simulink model "vspu2024_model"  (R2022b)
settings: Solver=ode1  StartTime=0.0  StopTime=25  FixedStep=10^-5  RelTol=1e-3
values from neighbouring files (symbols this model uses):
  a0 = 1    [vspu_params.m]
  a1 = 2    [vspu_params.m]
  a2 = 1    [vspu_params.m]
  a3 = 2    [vspu_params.m]
  a4 = 0.01    [vspu_params.m]
  a5 = 1    [vspu_params.m]
  a6 = 1    [vspu_params.m]
  a7 = 1    [vspu_params.m]
  k = 1    [vspu_params.m]
undefined symbols (not defined in the file or in its folder): adjoint
settings Model: Creator=LastConst  LastModifiedBy=LastConst
settings SolverCC: AlgebraicLoopSolver=TrustRegion
settings DataIOCC: ReturnWorkspaceOutputs=off
settings DebuggingCC: UnconnectedInputMsg=warning  UnconnectedOutputMsg=warning  UnconnectedLineMsg=warning  SFMachineParentedDataDiag=warning  ArithmeticOperatorsInVariantConditions=warning
settings ModelReferenceCC: EnableRefExpFcnMdlSchedulingChecks=on
settings SFSimCC: SimUseLocalCustomCode=off  CustomCodeUndefinedFunction=UseInterfaceOnly
settings RTWCC: RTWUseLocalCustomCode=off
settings CodeAppCC: StateflowObjectComments=on

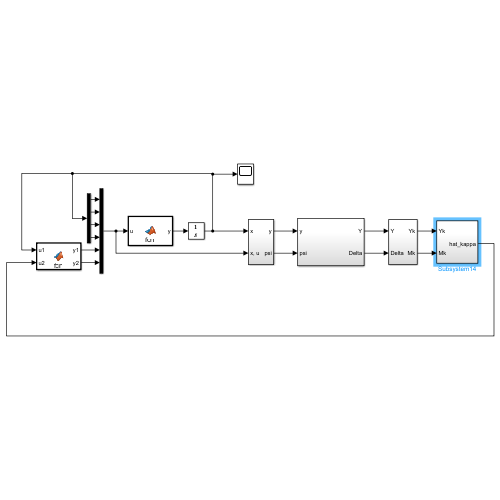
[thumbnail: Simulink's stored preview of the top-level diagram]
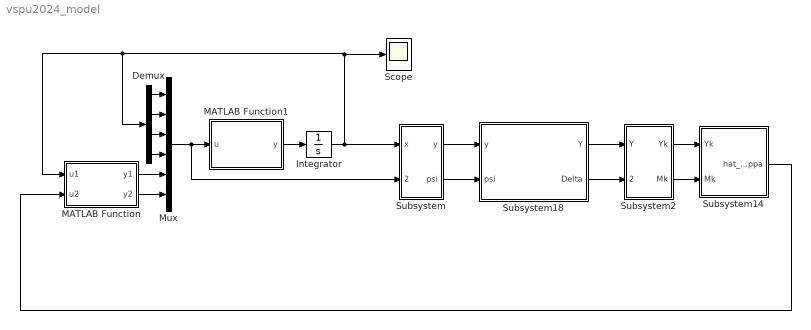
== system vspu2024_model ==
  Demux : Demux
  Integrator : Integrator  InitialCondition=[-1; 1;0.2;-0.2]*100
  MATLAB Function : MATLAB Function  TreatAsAtomicUnit=on
  MATLAB Function1 : MATLAB Function  TreatAsAtomicUnit=on
  Mux : Mux  Inputs=6
  Scope : Scope
  Subsystem : Subsystem
  Subsystem14 : Subsystem
  Subsystem18 : Subsystem
  Subsystem2 : Subsystem
  wires:
  Demux/1 -> Mux/1
  Demux/2 -> Mux/2
  Demux/3 -> Mux/3
  Demux/4 -> Mux/4
  MATLAB Function/2(y2) -> Mux/6
  MATLAB Function/1(y1) -> Mux/5
  Integrator/1 -> Scope/1, MATLAB Function/1(u1), Demux/1, Subsystem/1(x)
  Subsystem14/1(hat_kappa) -> MATLAB Function/2(u2)
  Mux/1 -> MATLAB Function1/1(u), Subsystem/2("x, u")
  MATLAB Function1/1(y) -> Integrator/1
  Subsystem2/1(Yk) -> Subsystem14/1(Yk)
  Subsystem2/2(Mk) -> Subsystem14/2(Mk)
  Subsystem/1(y) -> Subsystem18/1(y)
  Subsystem/2(psi) -> Subsystem18/2(psi)
  Subsystem18/1(Y) -> Subsystem2/1(Y)
  Subsystem18/2(Delta) -> Subsystem2/2(Delta)

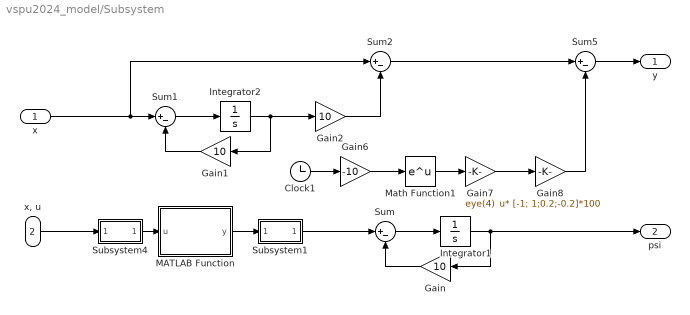
== system vspu2024_model/Subsystem ==
  x : Inport
  "x, u" : Inport  Port=2
  Clock1 : Clock
  Gain : Gain  Gain=10
  Gain1 : Gain  Gain=10
  Gain2 : Gain  Gain=10
  Gain6 : Gain  Gain=-10
  Gain7 : Gain  Gain=eye(4)
  Gain8 : Gain  Gain=[-1; 1;0.2;-0.2]*100  Multiplication=Matrix(u*K)
  Integrator1 : Integrator
  Integrator2 : Integrator
  MATLAB Function : MATLAB Function  TreatAsAtomicUnit=on
  Math Function1 : Math  SignedPower=on
  Subsystem1 : Subsystem
  Subsystem4 : Subsystem
  Sum{,1..2,5} (4 alike) : Sum  Inputs=|+-
  y : Outport
  psi : Outport  Port=2
  wires:
  MATLAB Function/1(y) -> Subsystem1/1(In1)
  Gain2/1 -> Sum2/2
  Sum/1 -> Integrator1/1
  Gain/1 -> Sum/2
  Sum1/1 -> Integrator2/1
  Integrator2/1 -> Gain2/1, Gain1/1
  Gain1/1 -> Sum1/2
  x/1 -> Sum2/1, Sum1/1
  "x, u"/1 -> Subsystem4/1(In1)
  Integrator1/1 -> psi/1, Gain/1
  Subsystem4/1(Out1) -> MATLAB Function/1(u)
  Subsystem1/1(Out1) -> Sum/1
  Gain6/1 -> Math Function1/1
  Clock1/1 -> Gain6/1
  Math Function1/1 -> Gain7/1
  Gain7/1 -> Gain8/1
  Gain8/1 -> Sum5/2
  Sum2/1 -> Sum5/1
  Sum5/1 -> y/1

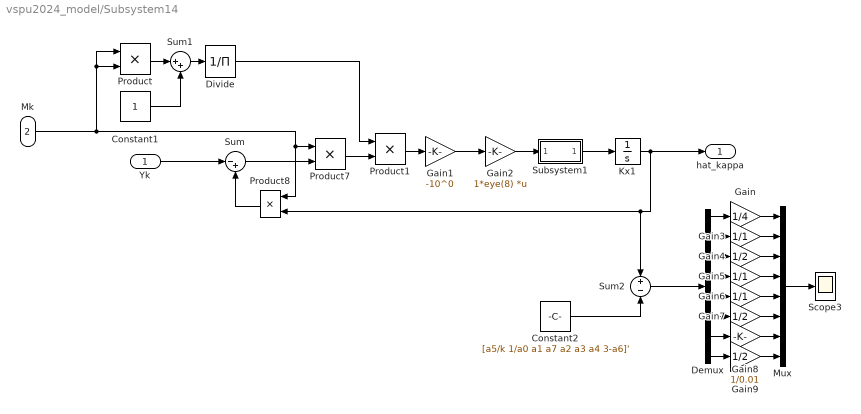
== system vspu2024_model/Subsystem14 ==
  Yk : Inport
  Mk : Inport  Port=2
  Constant1 : Constant
  Constant2 : Constant  Value=[a5/k 1/a0 a1 a7 a2 a3 a4 3-a6]'
  Demux : Demux  Outputs=8
  Divide : Product  Inputs=/
  Gain : Gain  Gain=1/4
  Gain1 : Gain  Gain=-10^0
  Gain2 : Gain  Gain=1*eye(8)  Multiplication=Matrix(K*u)
  Gain3 : Gain  Gain=1/1
  Gain4 : Gain  Gain=1/2
  Gain5 : Gain  Gain=1/1
  Gain6 : Gain  Gain=1/1
  Gain7 : Gain  Gain=1/2
  Gain8 : Gain  Gain=1/0.01
  Gain9 : Gain  Gain=1/2
  Kx1 : Integrator  InitialCondition=[5 0 0 0 0 0 0 0]'
  Mux : Mux  Inputs=8
  Product{,1,7..8} (4 alike) : Product
  Scope3 : Scope
  Subsystem1 : Subsystem
  Sum : Sum  Inputs=|-+
  Sum1 : Sum  Inputs=|++
  Sum2 : Sum  Inputs=+-
  hat_kappa : Outport
  wires:
  Product8/1 -> Sum/2
  Product7/1 -> Product1/2
  Sum/1 -> Product7/2
  Divide/1 -> Product1/1
  Subsystem1/1(Out1) -> Kx1/1
  Product1/1 -> Gain1/1
  Yk/1 -> Sum/1
  Gain2/1 -> Subsystem1/1(In1)
  Mk/1 -> Product/1, Product/2, Product7/1, Product8/1
  Kx1/1 -> hat_kappa/1, Sum2/1, Product8/2
  Constant2/1 -> Sum2/2
  Sum1/1 -> Divide/1
  Product/1 -> Sum1/1
  Constant1/1 -> Sum1/2
  Gain1/1 -> Gain2/1
  Sum2/1 -> Demux/1
  Mux/1 -> Scope3/1
  Demux/3 -> Gain4/1
  Demux/1 -> Gain/1
  Demux/2 -> Gain3/1
  Demux/4 -> Gain5/1
  Demux/5 -> Gain6/1
  Demux/6 -> Gain7/1
  Demux/7 -> Gain8/1
  Demux/8 -> Gain9/1
  Gain/1 -> Mux/1
  Gain3/1 -> Mux/2
  Gain4/1 -> Mux/3
  Gain5/1 -> Mux/4
  Gain6/1 -> Mux/5
  Gain7/1 -> Mux/6
  Gain8/1 -> Mux/7
  Gain9/1 -> Mux/8

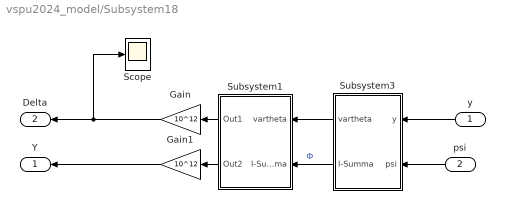
== system vspu2024_model/Subsystem18 ==
  y : Inport
  psi : Inport  Port=2
  Gain : Gain  Gain=10^12
  Gain1 : Gain  Gain=10^12
  Scope : Scope
  Subsystem1 : Subsystem
  Subsystem3 : Subsystem
  Y : Outport
  Delta : Outport  Port=2
  wires:
  Subsystem1/2(Out2) -> Gain1/1
  y/1 -> Subsystem3/1(y)
  Subsystem3/2(I-Summa) -> Subsystem1/2(I-Summa)  "Ф"
  Gain/1 -> Scope/1, Delta/1
  Subsystem3/1(vartheta) -> Subsystem1/1(vartheta)
  Gain1/1 -> Y/1
  Subsystem1/1(Out1) -> Gain/1
  psi/1 -> Subsystem3/2(psi)

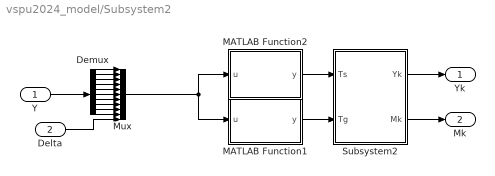
== system vspu2024_model/Subsystem2 ==
  Y : Inport
  Delta : Inport  Port=2
  Demux : Demux  Outputs=10
  MATLAB Function1 : MATLAB Function  TreatAsAtomicUnit=on
  MATLAB Function2 : MATLAB Function  TreatAsAtomicUnit=on
  Mux : Mux  Inputs=11
  Subsystem2 : Subsystem
  Yk : Outport
  Mk : Outport  Port=2
  wires:
  MATLAB Function2/1(y) -> Subsystem2/1(Ts)
  MATLAB Function1/1(y) -> Subsystem2/2(Tg)
  Y/1 -> Demux/1
  Mux/1 -> MATLAB Function2/1(u), MATLAB Function1/1(u)
  Subsystem2/2(Mk) -> Mk/1
  Subsystem2/1(Yk) -> Yk/1
  Demux/1 -> Mux/1
  Demux/2 -> Mux/2
  Demux/3 -> Mux/3
  Demux/4 -> Mux/4
  Demux/5 -> Mux/5
  Demux/6 -> Mux/6
  Demux/7 -> Mux/7
  Demux/8 -> Mux/8
  Demux/9 -> Mux/9
  Demux/10 -> Mux/10
  Delta/1 -> Mux/11

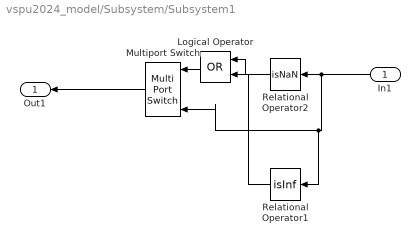
== system vspu2024_model/Subsystem/Subsystem1 ==
  In1 : Inport
  Logical Operator : Logic  Operator=OR  AllPortsSameDT=off  OutDataTypeStr=boolean
  Multiport Switch : MultiPortSwitch  DataPortOrder=Specify indices  DataPortIndices={1,0}  SaturateOnIntegerOverflow=off  InputSameDT=off
  Relational Operator1 : RelationalOperator  Operator=isInf  OutDataTypeStr=boolean  RndMeth=Simplest  InputSameDT=off
  Relational Operator2 : RelationalOperator  Operator=isNaN  OutDataTypeStr=boolean  RndMeth=Simplest  InputSameDT=off
  Out1 : Outport
  wires:
  Relational Operator2/1 -> Logical Operator/1
  In1/1 -> Relational Operator2/1, Relational Operator1/1, Multiport Switch/3
  Multiport Switch/1 -> Out1/1
  Logical Operator/1 -> Multiport Switch/1
  Relational Operator1/1 -> Logical Operator/2

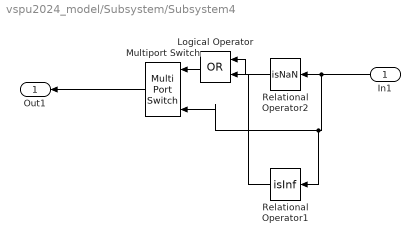
== system vspu2024_model/Subsystem/Subsystem4 ==
  In1 : Inport
  Logical Operator : Logic  Operator=OR  AllPortsSameDT=off  OutDataTypeStr=boolean
  Multiport Switch : MultiPortSwitch  DataPortOrder=Specify indices  DataPortIndices={1,0}  SaturateOnIntegerOverflow=off  InputSameDT=off
  Relational Operator1 : RelationalOperator  Operator=isInf  OutDataTypeStr=boolean  RndMeth=Simplest  InputSameDT=off
  Relational Operator2 : RelationalOperator  Operator=isNaN  OutDataTypeStr=boolean  RndMeth=Simplest  InputSameDT=off
  Out1 : Outport
  wires:
  Relational Operator2/1 -> Logical Operator/1
  In1/1 -> Relational Operator2/1, Relational Operator1/1, Multiport Switch/3
  Multiport Switch/1 -> Out1/1
  Logical Operator/1 -> Multiport Switch/1
  Relational Operator1/1 -> Logical Operator/2

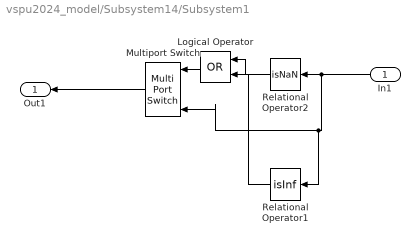
== system vspu2024_model/Subsystem14/Subsystem1 ==
  In1 : Inport
  Logical Operator : Logic  Operator=OR  AllPortsSameDT=off  OutDataTypeStr=boolean
  Multiport Switch : MultiPortSwitch  DataPortOrder=Specify indices  DataPortIndices={1,0}  SaturateOnIntegerOverflow=off  InputSameDT=off
  Relational Operator1 : RelationalOperator  Operator=isInf  OutDataTypeStr=boolean  RndMeth=Simplest  InputSameDT=off
  Relational Operator2 : RelationalOperator  Operator=isNaN  OutDataTypeStr=boolean  RndMeth=Simplest  InputSameDT=off
  Out1 : Outport
  wires:
  Relational Operator1/1 -> Logical Operator/2
  Logical Operator/1 -> Multiport Switch/1
  Multiport Switch/1 -> Out1/1
  In1/1 -> Multiport Switch/3, Relational Operator1/1, Relational Operator2/1
  Relational Operator2/1 -> Logical Operator/1

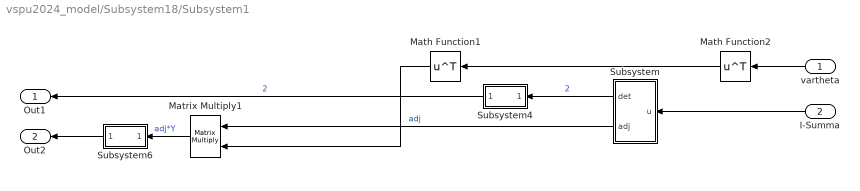
== system vspu2024_model/Subsystem18/Subsystem1 ==
  vartheta : Inport
  I-Summa : Inport  Port=2
  Math Function1 : Math  Operator=transpose  SignedPower=on
  Math Function2 : Math  Operator=transpose  SignedPower=on
  Matrix Multiply1 : Product  Multiplication=Matrix(*)
  Subsystem : Subsystem
  Subsystem4 : Subsystem
  Subsystem6 : Subsystem
  Out1 : Outport
  Out2 : Outport  Port=2
  wires:
  I-Summa/1 -> Subsystem/1(u)
  Subsystem/1(det) -> Subsystem4/1(In1)  "2"
  Subsystem4/1(Out1) -> Out1/1  "2"
  vartheta/1 -> Math Function2/1
  Subsystem6/1(Out1) -> Out2/1
  Subsystem/2(adj) -> Matrix Multiply1/1  "adj"
  Math Function1/1 -> Matrix Multiply1/2
  Matrix Multiply1/1 -> Subsystem6/1(In1)  "adj*Y"
  Math Function2/1 -> Math Function1/1

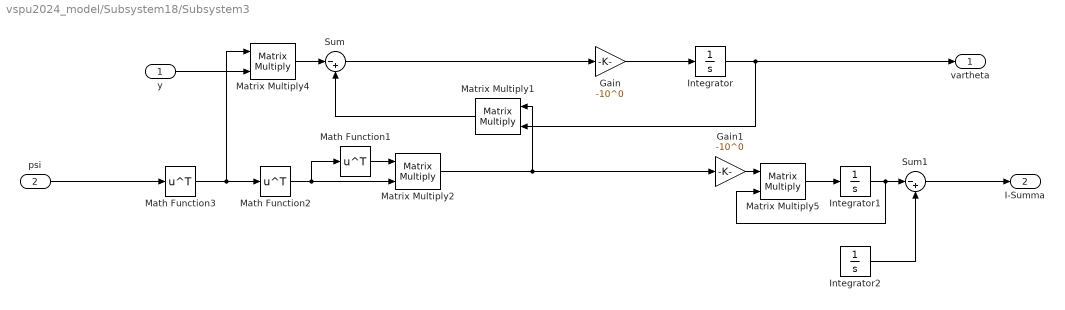
== system vspu2024_model/Subsystem18/Subsystem3 ==
  y : Inport
  psi : Inport  Port=2
  Gain : Gain  Gain=-10^0
  Gain1 : Gain  Gain=-10^0
  Integrator : Integrator  InitialCondition=zeros(10,1)
  Integrator1 : Integrator  InitialCondition=eye(10)
  Integrator2 : Integrator  InitialCondition=eye(10)
  Math Function1 : Math  Operator=transpose
  Math Function2 : Math  Operator=transpose
  Math Function3 : Math  Operator=transpose
  Matrix Multiply{1..2,4..5} (4 alike) : Product  Multiplication=Matrix(*)
  Sum : Sum  Inputs=|-+
  Sum1 : Sum  Inputs=|-+
  vartheta : Outport
  I-Summa : Outport  Port=2
  wires:
  y/1 -> Matrix Multiply4/2
  Sum/1 -> Gain/1
  Integrator1/1 -> Matrix Multiply5/2, Sum1/1
  Gain1/1 -> Matrix Multiply5/1
  Matrix Multiply2/1 -> Gain1/1, Matrix Multiply1/1
  Math Function1/1 -> Matrix Multiply2/1
  psi/1 -> Math Function3/1
  Gain/1 -> Integrator/1
  Integrator2/1 -> Sum1/2
  Sum1/1 -> I-Summa/1
  Integrator/1 -> Matrix Multiply1/2, vartheta/1
  Matrix Multiply1/1 -> Sum/2
  Matrix Multiply4/1 -> Sum/1
  Math Function3/1 -> Matrix Multiply4/1, Math Function2/1
  Matrix Multiply5/1 -> Integrator1/1
  Math Function2/1 -> Math Function1/1, Matrix Multiply2/2

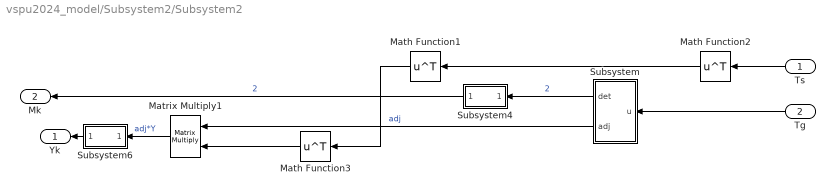
== system vspu2024_model/Subsystem2/Subsystem2 ==
  Ts : Inport
  Tg : Inport  Port=2
  Math Function1 : Math  Operator=transpose  SignedPower=on
  Math Function2 : Math  Operator=transpose  SignedPower=on
  Math Function3 : Math  Operator=transpose  SignedPower=on
  Matrix Multiply1 : Product  Multiplication=Matrix(*)
  Subsystem : Subsystem
  Subsystem4 : Subsystem
  Subsystem6 : Subsystem
  Yk : Outport
  Mk : Outport  Port=2
  wires:
  Tg/1 -> Subsystem/1(u)
  Subsystem/1(det) -> Subsystem4/1(In1)  "2"
  Subsystem4/1(Out1) -> Mk/1  "2"
  Ts/1 -> Math Function2/1
  Subsystem6/1(Out1) -> Yk/1
  Subsystem/2(adj) -> Matrix Multiply1/1  "adj"
  Math Function1/1 -> Math Function3/1
  Matrix Multiply1/1 -> Subsystem6/1(In1)  "adj*Y"
  Math Function2/1 -> Math Function1/1
  Math Function3/1 -> Matrix Multiply1/2

== system vspu2024_model/Subsystem18/Subsystem1/Subsystem ==
  u : Inport
  Interpreted MATLAB Function : MATLABFcn  MATLABFcn=adjoint(u)  Output1D=off
  MATLAB Function : MATLAB Function  TreatAsAtomicUnit=on
  det : Outport
  adj : Outport  Port=2
  wires:
  Interpreted MATLAB Function/1 -> adj/1
  MATLAB Function/1(y) -> det/1
  u/1 -> Interpreted MATLAB Function/1, MATLAB Function/1(u)

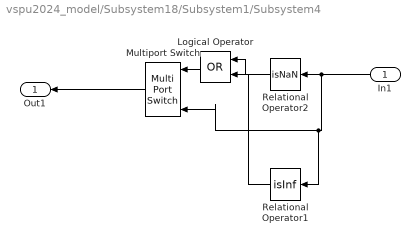
== system vspu2024_model/Subsystem18/Subsystem1/Subsystem4 ==
  In1 : Inport
  Logical Operator : Logic  Operator=OR  AllPortsSameDT=off  OutDataTypeStr=boolean
  Multiport Switch : MultiPortSwitch  DataPortOrder=Specify indices  DataPortIndices={1,0}  SaturateOnIntegerOverflow=off  InputSameDT=off
  Relational Operator1 : RelationalOperator  Operator=isInf  OutDataTypeStr=boolean  RndMeth=Simplest  InputSameDT=off
  Relational Operator2 : RelationalOperator  Operator=isNaN  OutDataTypeStr=boolean  RndMeth=Simplest  InputSameDT=off
  Out1 : Outport
  wires:
  Relational Operator2/1 -> Logical Operator/1
  In1/1 -> Relational Operator2/1, Relational Operator1/1, Multiport Switch/3
  Multiport Switch/1 -> Out1/1
  Logical Operator/1 -> Multiport Switch/1
  Relational Operator1/1 -> Logical Operator/2

== system vspu2024_model/Subsystem18/Subsystem1/Subsystem6 ==
  In1 : Inport
  Logical Operator : Logic  Operator=OR  AllPortsSameDT=off  OutDataTypeStr=boolean
  Multiport Switch : MultiPortSwitch  DataPortOrder=Specify indices  DataPortIndices={1,0}  SaturateOnIntegerOverflow=off  InputSameDT=off
  Relational Operator1 : RelationalOperator  Operator=isInf  OutDataTypeStr=boolean  RndMeth=Simplest  InputSameDT=off
  Relational Operator2 : RelationalOperator  Operator=isNaN  OutDataTypeStr=boolean  RndMeth=Simplest  InputSameDT=off
  Out1 : Outport
  wires:
  Relational Operator2/1 -> Logical Operator/1
  In1/1 -> Relational Operator2/1, Relational Operator1/1, Multiport Switch/3
  Multiport Switch/1 -> Out1/1
  Logical Operator/1 -> Multiport Switch/1
  Relational Operator1/1 -> Logical Operator/2

== system vspu2024_model/Subsystem2/Subsystem2/Subsystem ==
  u : Inport
  Interpreted MATLAB Function : MATLABFcn  MATLABFcn=adjoint(u)  Output1D=off
  MATLAB Function : MATLAB Function  TreatAsAtomicUnit=on
  det : Outport
  adj : Outport  Port=2
  wires:
  Interpreted MATLAB Function/1 -> adj/1
  MATLAB Function/1(y) -> det/1
  u/1 -> Interpreted MATLAB Function/1, MATLAB Function/1(u)

== system vspu2024_model/Subsystem2/Subsystem2/Subsystem4 ==
  In1 : Inport
  Logical Operator : Logic  Operator=OR  AllPortsSameDT=off  OutDataTypeStr=boolean
  Multiport Switch : MultiPortSwitch  DataPortOrder=Specify indices  DataPortIndices={1,0}  SaturateOnIntegerOverflow=off  InputSameDT=off
  Relational Operator1 : RelationalOperator  Operator=isInf  OutDataTypeStr=boolean  RndMeth=Simplest  InputSameDT=off
  Relational Operator2 : RelationalOperator  Operator=isNaN  OutDataTypeStr=boolean  RndMeth=Simplest  InputSameDT=off
  Out1 : Outport
  wires:
  Relational Operator2/1 -> Logical Operator/1
  In1/1 -> Relational Operator2/1, Relational Operator1/1, Multiport Switch/3
  Multiport Switch/1 -> Out1/1
  Logical Operator/1 -> Multiport Switch/1
  Relational Operator1/1 -> Logical Operator/2

== system vspu2024_model/Subsystem2/Subsystem2/Subsystem6 ==
  In1 : Inport
  Logical Operator : Logic  Operator=OR  AllPortsSameDT=off  OutDataTypeStr=boolean
  Multiport Switch : MultiPortSwitch  DataPortOrder=Specify indices  DataPortIndices={1,0}  SaturateOnIntegerOverflow=off  InputSameDT=off
  Relational Operator1 : RelationalOperator  Operator=isInf  OutDataTypeStr=boolean  RndMeth=Simplest  InputSameDT=off
  Relational Operator2 : RelationalOperator  Operator=isNaN  OutDataTypeStr=boolean  RndMeth=Simplest  InputSameDT=off
  Out1 : Outport
  wires:
  Relational Operator2/1 -> Logical Operator/1
  In1/1 -> Relational Operator2/1, Relational Operator1/1, Multiport Switch/3
  Multiport Switch/1 -> Out1/1
  Logical Operator/1 -> Multiport Switch/1
  Relational Operator1/1 -> Logical Operator/2

== matlab function vspu2024_model/Subsystem18/Subsystem1/Subsystem/MATLAB Function ==
  data: u input; y output
function y = fcn(u)

y = det(u);

== matlab function vspu2024_model/MATLAB Function1 ==
  data: u input; y output
function y = fcn(u)
a0=1;
a1=2;
a2=1;
a3=2;
a4=0.01;
a5=1;
k=1;
a6=1;
a7=1;
y = [u(2); a0*u(4)-a1*sin(u(1))-(a2+a3*sin(u(1)))*u(3)-a4*u(3)^2; -k*u(3)+a5*sin(u(1))*u(2)+k*u(5); -a6*u(4)-a7*u(2)+u(6)];

== matlab function vspu2024_model/Subsystem/MATLAB Function ==
  data: u input; y output
function y = fcn(u)

y = [u(2) 0 0 0 0 0 0 0 0 0;
 0 u(4) -sin(u(1)) -u(3) -sin(u(1))*u(3) -u(3)*u(3) 0 0 0 0;
 0 0 0 0 0 0 -u(3)+u(5) u(2)*sin(u(1)) 0 0;
 u(6) 0 0 0 0 0 0 0 -u(4) -u(2)];;

== matlab function vspu2024_model/Subsystem2/MATLAB Function1 ==
  data: u input; y output
function y = fcn(u)
y = diag([u(7) u(2)*u(2) u(11)*ones(1,6)]);

== matlab function vspu2024_model/Subsystem2/MATLAB Function2 ==
  data: u input; y output
function y = fcn(u)
y = [u(8) u(11)*u(2) u(3) u(10) u(4) u(5) u(6) 3*u(11)-u(9)];

== matlab function vspu2024_model/Subsystem2/Subsystem2/Subsystem/MATLAB Function ==
  data: u input; y output
function y = fcn(u)

y = det(u);

== matlab function vspu2024_model/MATLAB Function ==
  data: u1 input; y1 output; u2 input; y2 output
function [y1, y2] = fcn(u1, u2)


y2 = -u2(2)*u1(1)+3*u2(3)*sin(u1(1))-u2(2)*3*u1(2)-u2(4)*u2(2)*u1(2)-u2(3)*cos(u1(1))*u1(2)+2*u2(2)*u2(5)*u1(3)+2*u2(6)*u2(2)*sin(u1(1))*u1(3)+2*u2(7)*u2(2)*u1(3)*u1(3)-u2(8)*u1(4);
y1 = -1*u2(1)*sin(u1(1))*u1(2);
